simulink model "Two5s2p"  (R2024a)
settings: Solver=VariableStepAuto  StartTime=0.0  StopTime=29000  RelTol=1e-3
libraries: fl_lib x32, nesl_utility x32, batteryecm_lib x10, BatteryCurrentManagement x1, BatteryBalancing x1
(part 1 of 3)
settings Model: Creator=ACER  LastModifiedBy=ACER

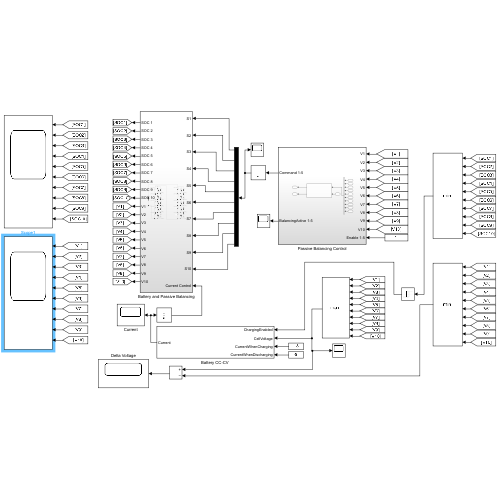
[thumbnail: Simulink's stored preview of the top-level diagram]
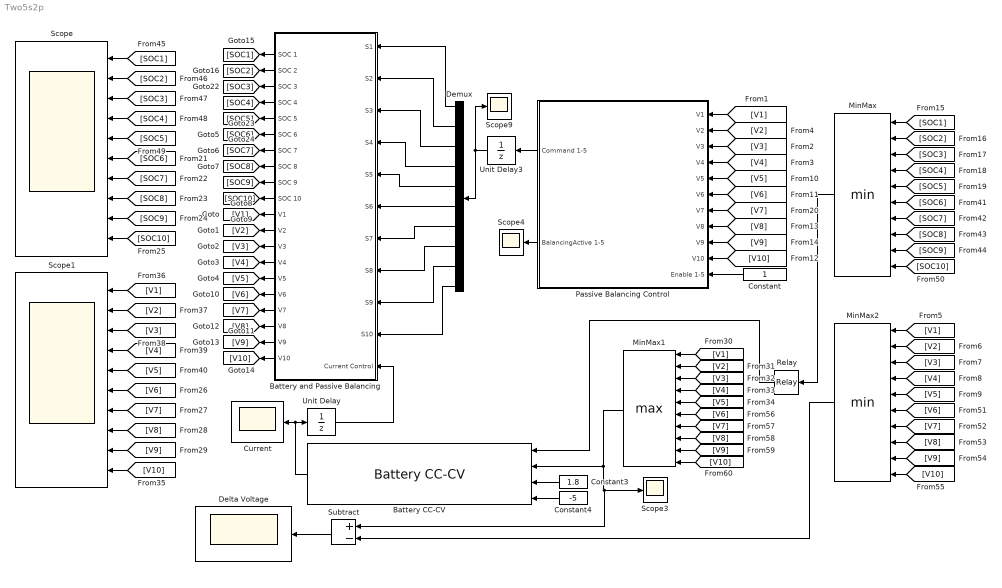
== system Two5s2p ==
  "Battery CC-CV " : BatteryCurrentManagement/Battery CC-CV  MaxCellVoltage=4.19  Kp=100  Ki=10  Kaw=1  Kt=1  Ts=1
      settings: LibrarySourceBlock=batt_sl_lib/Current Management/Battery CC-CV
  Battery and Passive Balancing : Subsystem
  Constant : Constant
  Constant3 : Constant  Value=1.8
  Constant4 : Constant  Value=-5
  Current : Scope
  Delta Voltage : Scope
  Demux : Demux  Outputs=10
  MinMax : MinMax  Inputs=10
  MinMax1 : MinMax  Function=max  Inputs=10
  MinMax2 : MinMax  Inputs=10
  Passive Balancing Control : Subsystem
  Relay : Relay  OnSwitchValue=0.990  OffSwitchValue=0.5  OnOutputValue=0  OffOutputValue=1
  Scope : Scope  NumInputPorts=10
  Scope1 : Scope  NumInputPorts=10
  Scope3 : Scope
  Scope4 : Scope
  Scope9 : Scope
  Subtract : Sum  Inputs=+-
  Unit Delay : UnitDelay  SampleTime=-1  HasFrameUpgradeWarning=on
  Unit Delay3 : UnitDelay  SampleTime=-1  HasFrameUpgradeWarning=on
  wires:
  MinMax2/1 -> Subtract/2
  Constant/1 -> Passive Balancing Control/11(Enable 1-5)
  Constant3/1 -> "Battery CC-CV "/3
  Subtract/1 -> Delta Voltage/1
  MinMax/1 -> Relay/1
  MinMax1/1 -> Subtract/1, Scope3/1, "Battery CC-CV "/2
  Relay/1 -> "Battery CC-CV "/1
  Passive Balancing Control/2(BalancingActive 1-5) -> Scope4/1
  Unit Delay3/1 -> Scope9/1, Demux/1
  Passive Balancing Control/1(Command 1-5) -> Unit Delay3/1
  Constant4/1 -> "Battery CC-CV "/4
  [V1] -> Passive Balancing Control/1(V1)
  [V2] -> Passive Balancing Control/2(V2)
  [V3] -> Passive Balancing Control/3(V3)
  [V4] -> Passive Balancing Control/4(V4)
  [V5] -> Passive Balancing Control/5(V5)
  [V6] -> Passive Balancing Control/6(V6)
  [V7] -> Passive Balancing Control/7(V7)
  [V8] -> Passive Balancing Control/8(V8)
  [V9] -> Passive Balancing Control/9(V9)
  [V10] -> Passive Balancing Control/10(V10)
  Demux/10 -> Battery and Passive Balancing/10(S10)
  Demux/9 -> Battery and Passive Balancing/9(S9)
  Demux/8 -> Battery and Passive Balancing/8(S8)
  Demux/7 -> Battery and Passive Balancing/7(S7)
  Demux/6 -> Battery and Passive Balancing/6(S6)
  Demux/1 -> Battery and Passive Balancing/1(S1)
  Demux/2 -> Battery and Passive Balancing/2(S2)
  Demux/3 -> Battery and Passive Balancing/3(S3)
  Demux/4 -> Battery and Passive Balancing/4(S4)
  Demux/5 -> Battery and Passive Balancing/5(S5)
  Battery and Passive Balancing/1(SOC 1) -> [SOC1]
  Battery and Passive Balancing/2(SOC 2) -> [SOC2]
  Battery and Passive Balancing/3(SOC 3) -> [SOC3]
  Battery and Passive Balancing/4(SOC 4) -> [SOC4]
  Battery and Passive Balancing/5(SOC 5) -> [SOC5]
  Battery and Passive Balancing/6(SOC 6) -> [SOC6]
  Battery and Passive Balancing/7(SOC 7) -> [SOC7]
  Battery and Passive Balancing/8(SOC 8) -> [SOC8]
  Battery and Passive Balancing/9(SOC 9) -> [SOC9]
  Battery and Passive Balancing/10(SOC 10) -> [SOC10]
  Battery and Passive Balancing/11(V1) -> [V1]
  Battery and Passive Balancing/12(V2) -> [V2]
  Battery and Passive Balancing/13(V3) -> [V3]
  Battery and Passive Balancing/14(V4) -> [V4]
  Battery and Passive Balancing/15(V5) -> [V5]
  Battery and Passive Balancing/16(V6) -> [V6]
  Battery and Passive Balancing/17(V7) -> [V7]
  Battery and Passive Balancing/18(V8) -> [V8]
  Battery and Passive Balancing/19(V9) -> [V9]
  Battery and Passive Balancing/20(V10) -> [V10]
  [SOC1] -> Scope/1
  [SOC2] -> Scope/2
  [SOC3] -> Scope/3
  [SOC4] -> Scope/4
  [SOC5] -> Scope/5
  [SOC6] -> Scope/6
  [SOC7] -> Scope/7
  [SOC8] -> Scope/8
  [SOC9] -> Scope/9
  [SOC10] -> Scope/10
  [V10] -> Scope1/10
  [V9] -> Scope1/9
  [V8] -> Scope1/8
  [V7] -> Scope1/7
  [V6] -> Scope1/6
  [V5] -> Scope1/5
  [V4] -> Scope1/4
  [V3] -> Scope1/3
  [V2] -> Scope1/2
  [V1] -> Scope1/1
  [V1] -> MinMax2/1
  [V2] -> MinMax2/2
  [V3] -> MinMax2/3
  [V4] -> MinMax2/4
  [V5] -> MinMax2/5
  [V6] -> MinMax2/6
  [V7] -> MinMax2/7
  [V8] -> MinMax2/8
  [V9] -> MinMax2/9
  [V10] -> MinMax2/10
  [SOC10] -> MinMax/10
  [SOC9] -> MinMax/9
  [SOC8] -> MinMax/8
  [SOC7] -> MinMax/7
  [SOC6] -> MinMax/6
  [SOC5] -> MinMax/5
  [SOC4] -> MinMax/4
  [SOC3] -> MinMax/3
  [SOC2] -> MinMax/2
  [SOC1] -> MinMax/1
  "Battery CC-CV "/1 -> Current/1, Unit Delay/1
  Unit Delay/1 -> Battery and Passive Balancing/11(Current Control)
  [V1] -> MinMax1/1
  [V2] -> MinMax1/2
  [V3] -> MinMax1/3
  [V4] -> MinMax1/4
  [V5] -> MinMax1/5
  [V7] -> MinMax1/7
  [V6] -> MinMax1/6
  [V8] -> MinMax1/8
  [V9] -> MinMax1/9
  [V10] -> MinMax1/10
